simulink model "Hexacopter"  (R2017a)
settings: Solver=VariableStepAuto  StartTime=0.0  StopTime=10.0  RelTol=1e-3
values from neighbouring files (symbols this model uses):
  b = 3.13*exp(-5)    [Hexacopter_values.m]    (also in values.m)
  d = 7.5*exp(-7)    [values.m]
  g = 9.81    [values.m]
  Jxx = 7.5*10^-3    (= 0.0075)    [Hexacopter_values.m]    (also in values.m = 7.5*exp(-3))
  Jyy = 7.5*10^-3    (= 0.0075)    [Hexacopter_values.m]    (also in values.m = 7.5*exp(-3))
  Jzz = 1.3*10^-2    (= 0.013)    [Hexacopter_values.m]    (also in values.m = 1.3*exp(-2))
  Kfax = 0.1    [Hexacopter_values.m]    (also in values.m)
  Kfay = 0.1    [Hexacopter_values.m]    (also in values.m)
  Kfaz = 0.15    [Hexacopter_values.m]    (also in values.m)
  Kftx = 1.5    [Hexacopter_values.m]
  Kfty = 0.1    [Hexacopter_values.m]
  Kftz = 1.9    [Hexacopter_values.m]
  l = 0.23    [Hexacopter_values.m]    (also in values.m = 1)
  m = 0.65    [Hexacopter_values.m]    (also in values.m = 5)
undefined symbols (not defined in the file or in its folder): i, J1, ux, uy
libraries: simulink x4
settings Model: Creator=Yash Shetye  LastModifiedBy=Jash

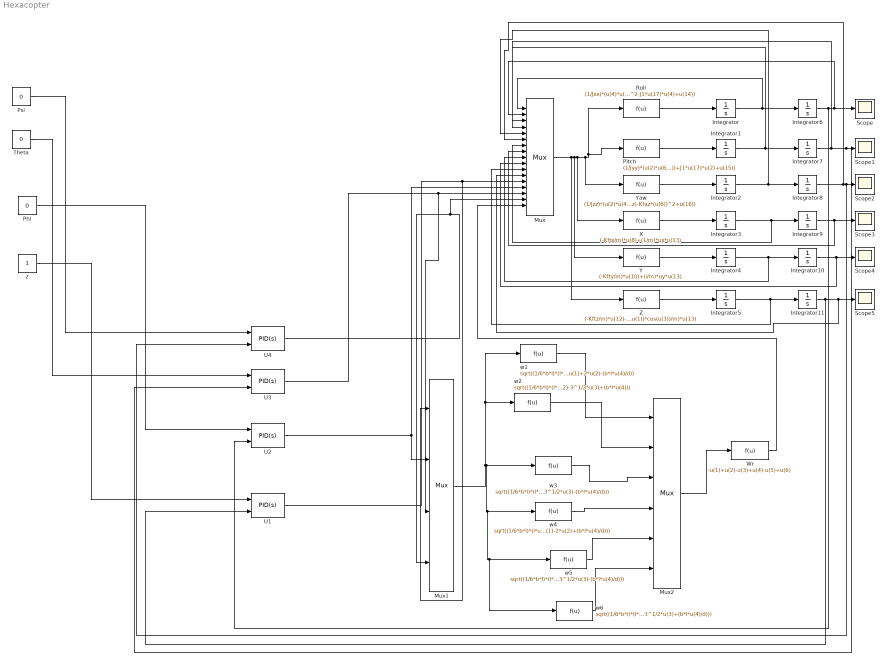
== system Hexacopter ==
  Integrator{,1..11} (12 alike) : Integrator
  Mux : Mux  Inputs=17
  Mux1 : Mux
  Mux2 : Mux  Inputs=6
  Phi : Constant  Value=0
  Pitch : Fcn  Expr=(1/Jyy)*(u(2)*u(6)*(Jzz-Jxx)-Kfay*(u(4)*u(4))+J1*u(17)*u(2)+u(15))
  Psi : Constant  Value=0
  Roll : Fcn  Expr=(1/Jxx)*(u(4)*u(6)*(Jyy-Jzz)-Kfax*(u(2))^2-J1*u(17)*u(4)+u(14))
  Scope{,1..5} (6 alike) : Scope
  Theta : Constant  Value=0
  U{1..4} (4 alike) : simulink/Continuous/PID Controller (2DOF)  Controller=PID  TimeDomain=Continuous-time  SampleTime=-1  IntegratorMethod=Forward Euler  FilterMethod=Forward Euler  Form=Parallel  UseFilter=on  ControllerParametersSource=internal  P=1  I=1  D=0  N=100  b=1  c=1  InitialConditionSource=internal  InitialConditionForIntegrator=0  InitialConditionForFilter=0  ExternalReset=none  LimitOutput=off  UpperSaturationLimit=inf  LowerSaturationLimit=-inf  LinearizeAsGain=on  AntiWindupMode=none  Kb=1  TrackingMode=off  Kt=1  PParamMin=[]  PParamMax=[]  IParamMin=[]  IParamMax=[]  DParamMin=[]  DParamMax=[]  NParamMin=[]  NParamMax=[]  bParamMin=[]  bParamMax=[]  cParamMin=[]  cParamMax=[]  KbParamMin=[]  KbParamMax=[]  KtParamMin=[]  KtParamMax=[]  POutMin=[]  POutMax=[]  IOutMin=[]  IOutMax=[]  DOutMin=[]  DOutMax=[]  NOutMin=[]  NOutMax=[]  bOutMin=[]  bOutMax=[]  cOutMin=[]  cOutMax=[]  KbOutMin=[]  KbOutMax=[]  KtOutMin=[]  KtOutMax=[]  IntegratorOutMin=[]  IntegratorOutMax=[]  FilterOutMin=[]  FilterOutMax=[]  SumOutMin=[]  SumOutMax=[]  Sum1OutMin=[]  Sum1OutMax=[]  Sum2OutMin=[]  Sum2OutMax=[]  Sum3OutMin=[]  Sum3OutMax=[]  SumI1OutMin=[]  SumI1OutMax=[]  SumI2OutMin=[]  SumI2OutMax=[]  SumI3OutMin=[]  SumI3OutMax=[]  SumDOutMin=[]  SumDOutMax=[]  SaturationOutMin=[]  SaturationOutMax=[]  IntegratorContinuousStateAttributes=''  IntegratorStateMustResolveToSignalObject=off  IntegratorRTWStateStorageClass=Auto  FilterContinuousStateAttributes=''  FilterStateMustResolveToSignalObject=off  FilterRTWStateStorageClass=Auto  DifferentiatorICPrevScaledInput=0  DifferentiatorOutMin=[]  DifferentiatorOutMax=[]  InitialConditionSetting=State (most efficient)
  Wr : Fcn  Expr=-u(1)+u(2)-u(3)+u(4)-u(5)+u(6)
  X : Fcn  Expr=(-Kftx/m)*u(8)+(1/m)*ux*u(13)
  Y : Fcn  Expr=(-Kfty/m)*u(10)+(i/m)*uy*u(13)
  Yaw : Fcn  Expr=(1/Jzz)*(u(2)*u(4)*(Jxx-Jzz)-Kfaz*(u(6))^2+u(16))
  Z : Fcn  Expr=(-Kftz/m)*u(12)-g+(cos(u(1))*cos(u(3))/m)*u(13)
  w1 : Fcn  Expr=sqrt((1/6*b*l)*(l*u(1)+2*u(2)-(b*l*u(4)/d))
  w2 : Fcn  Expr=sqrt((1/6*b*l)*(l*u(1)+u(2)-3^1/2*u(3)+(b*l*u(4)))
  w3 : Fcn  Expr=sqrt((1/6*b*l)*(l*u(1)-u(2)-3^1/2*u(3)-(b*l*u(4)/d)))
  w4 : Fcn  Expr=sqrt((1/6*b*l)*(l*u(1)-2*u(2)+(b*l*u(4)/d)))
  w5 : Fcn  Expr=sqrt((1/6*b*l)*(l*u(1)-u(2)+3^1/2*u(3)-(b*l*u(4)/d)))
  w6 : Fcn  Expr=sqrt((1/6*b*l)*(l*u(1)+u(2)+3^1/2*u(3)+(b*l*u(4)/d)))
  z : Constant
  wires:
  Roll/1 -> Integrator/1
  Mux/1 -> Z/1, Y/1, X/1, Yaw/1, Pitch/1, Roll/1
  Pitch/1 -> Integrator1/1
  Yaw/1 -> Integrator2/1
  X/1 -> Integrator3/1
  Y/1 -> Integrator4/1
  Z/1 -> Integrator5/1
  Integrator/1 -> Mux/1, Integrator6/1
  Integrator1/1 -> Mux/3, Integrator7/1
  Integrator3/1 -> Mux/7, Integrator9/1
  Integrator4/1 -> Mux/9, Integrator10/1
  Integrator5/1 -> Mux/11, Integrator11/1
  Integrator6/1 -> Mux/2, Scope/1, U2/2
  Integrator7/1 -> Mux/4, U3/2, Scope1/1
  Integrator8/1 -> U4/2, Scope2/1, Mux/6
  Integrator9/1 -> Mux/8, Scope3/1
  Integrator10/1 -> Mux/10, Scope4/1
  Integrator11/1 -> U1/2, Mux/12, Scope5/1
  U1/1 -> Mux1/1, Mux/13
  U2/1 -> Mux/14, Mux1/2
  U3/1 -> Mux1/3, Mux/15
  U4/1 -> Mux/16, Mux1/4
  Integrator2/1 -> Mux/5, Integrator8/1
  Psi/1 -> U4/1
  Theta/1 -> U3/1
  Phi/1 -> U2/1
  z/1 -> U1/1
  Mux1/1 -> w2/1, w1/1, w6/1, w5/1, w4/1, w3/1
  w1/1 -> Mux2/1
  w2/1 -> Mux2/2
  w3/1 -> Mux2/3
  w4/1 -> Mux2/4
  w5/1 -> Mux2/5
  w6/1 -> Mux2/6
  Mux2/1 -> Wr/1
  Wr/1 -> Mux/17
